simulink model "CombinatorialLogic_TestGen4"  (R2017b)
settings: Solver=FixedStepDiscrete  StartTime=0.0  StopTime=10.0  RelTol=1e-3
undefined symbols (not defined in the file): Block_TestLib, reset
settings Model: Creator=hbourbou  LastModifiedBy=hbourbou
settings DebuggingCC: ParameterOverflowMsg=none

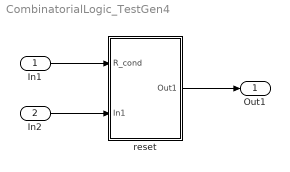
== system CombinatorialLogic_TestGen4 ==
  In1 : Inport
  In2 : Inport  Port=2
  reset : Subsystem  AncestorBlock=Block_TestLib/reset
  Out1 : Outport
  wires:
  In1/1 -> reset/1(R_cond)
  In2/1 -> reset/2(In1)
  reset/1(Out1) -> Out1/1

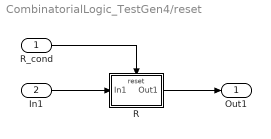
== system CombinatorialLogic_TestGen4/reset ==
  R_cond : Inport  OutDataTypeStr=boolean
  In1 : Inport  Port=2
  R : Subsystem  TreatAsAtomicUnit=on
  Out1 : Outport
  wires:
  R_cond/1 -> R/Reset
  In1/1 -> R/1(In1)
  R/1(Out1) -> Out1/1

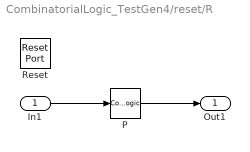
== system CombinatorialLogic_TestGen4/reset/R ==
  In1 : Inport  OutMin=0  OutMax=1  OutDataTypeStr=boolean
  Reset : ResetPort  DisableCoverage=on
  P : CombinatorialLogic  TruthTable=[0.425921001993938;0.747688815373207;0.743664792219808;0.83479433814678;0.703845037815539;0.603431275868441;0.434319098695933;0.13773593511635;0.690299870119745;0.602036754078748;0.851785416994308;0.270851275512656;0.964222367855326;0.151585308634602;0.0523980979325236;0.697014119613637]
  Out1 : Outport
  wires:
  In1/1 -> P/1
  P/1 -> Out1/1
